simulink model "untitled1"  (R2022b)
settings: Solver=FixedStepDiscrete  StartTime=0.0  StopTime=1  FixedStep=1  RelTol=1e-3
settings Model: Creator=vanch  LastModifiedBy=vanch

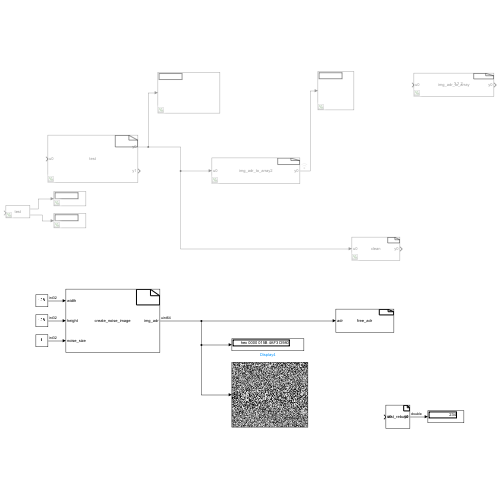
[thumbnail: Simulink's stored preview of the top-level diagram]
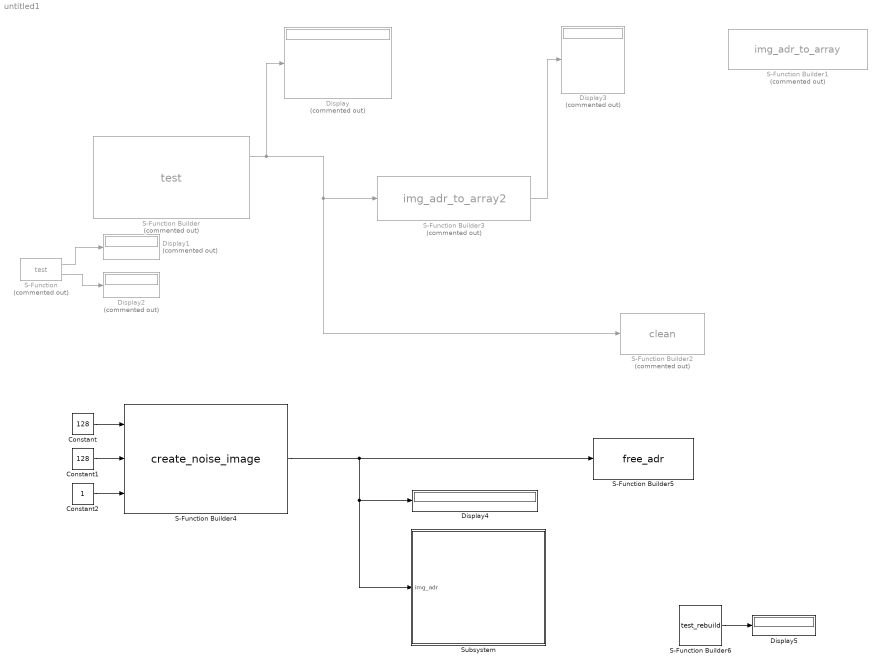
== system untitled1 ==
  Constant : Constant  Value=128  OutDataTypeStr=int32
  Constant1 : Constant  Value=128  OutDataTypeStr=int32
  Constant2 : Constant  OutDataTypeStr=int32
  Display{,1..3} (4 alike) : Display  Commented=on
      Display settings: Format=hex (Stored Integer)
  Display4 : Display
      settings: Format=hex (Stored Integer)
  Display5 : Display
  S-Function : S-Function  Commented=on  FunctionName=test  Parameters=3  SFunctionDeploymentMode=off  EnableBusSupport=off
  S-Function Builder : S-Function  Commented=on  FunctionName=test  Parameters=1  SFunctionModules=test_wrapper.cpp  SFunctionDeploymentMode=off  EnableBusSupport=off  mask(S-Function Builder){}
      mask help: Simulink:masks:SFunctionBuilder_MD
      mask init:
      | val = [[.9  0.75 0.75 1 1 .9 .9 1]',[1 1 0.75 0.75 .9 .9 1 .9]'];try , sys = get_param(gcb,'SfunBuilderFcnName');if isempty(sys), sys = get_param(gcb,'FunctionName'); end,catch, sys = get_param(gcb,'FunctionName'); end
      settings: CopyFcn=set_param(gcbh,'LinkStatus','none')  OpenFcn=sfunctionwizard(gcbh)
      mask Display:
      | plot(val(:,1),val(:,2))
      | disp(sys)
      | port_label('input',1,'u0')
      | port_label('output',1,'y0')
      | port_label('output',2,'y1')
  S-Function Builder1 : S-Function  Commented=on  FunctionName=img_adr_to_array  SFunctionModules=img_adr_to_array_wrapper.cpp  SFunctionDeploymentMode=off  EnableBusSupport=off  mask(S-Function Builder){}
      mask help: Simulink:masks:SFunctionBuilder_MD
      mask init: same as untitled1/S-Function Builder
      settings: CopyFcn=set_param(gcbh,'LinkStatus','none')  OpenFcn=sfunctionwizard(gcbh)
      mask Display: plot(val(:,1),val(:,2)),disp(sys),port_label('input',1,'u0'),port_label('output',1,'y0'),port_label('output',2,'y1')
  S-Function Builder2 : S-Function  Commented=on  FunctionName=clean  SFunctionModules=clean_wrapper.cpp  SFunctionDeploymentMode=off  EnableBusSupport=off  mask(S-Function Builder){}
      mask help: Simulink:masks:SFunctionBuilder_MD
      mask init: same as untitled1/S-Function Builder
      settings: CopyFcn=set_param(gcbh,'LinkStatus','none')  OpenFcn=sfunctionwizard(gcbh)
      mask Display:
      | plot(val(:,1),val(:,2))
      | disp(sys)
      | port_label('input',1,'u0')
      | port_label('output',1,'y0')
  S-Function Builder3 : S-Function  Commented=on  FunctionName=img_adr_to_array2  SFunctionModules=img_adr_to_array2_wrapper.cpp  SFunctionDeploymentMode=off  EnableBusSupport=off  mask(S-Function Builder){}
      mask help: Simulink:masks:SFunctionBuilder_MD
      mask init: same as untitled1/S-Function Builder
      settings: CopyFcn=set_param(gcbh,'LinkStatus','none')  OpenFcn=sfunctionwizard(gcbh)
      mask Display:
      | plot(val(:,1),val(:,2))
      | disp(sys)
      | port_label('input',1,'u0')
      | port_label('output',1,'y0')
  S-Function Builder4 : S-Function  FunctionName=create_noise_image  SFunctionModules=create_noise_image_wrapper.c  SFunctionDeploymentMode=off  EnableBusSupport=off  mask(S-Function Builder){}
      mask help: Simulink:masks:SFunctionBuilder_MD
      mask init: same as untitled1/S-Function Builder
      settings: CopyFcn=set_param(gcbh,'LinkStatus','none')  OpenFcn=sfunctionwizard(gcbh)
      mask Display:
      | plot(val(:,1),val(:,2))
      | disp(sys)
      | port_label('input',1,'width')
      | port_label('input',2,'height')
      | port_label('input',3,'noise_size')
      | port_label('output',1,'img_adr')
  S-Function Builder5 : S-Function  Priority=2  FunctionName=free_adr  SFunctionModules=free_adr_wrapper.c  SFunctionDeploymentMode=off  EnableBusSupport=off  mask(S-Function Builder){}
      mask help: Simulink:masks:SFunctionBuilder_MD
      mask init: same as untitled1/S-Function Builder
      settings: CopyFcn=set_param(gcbh,'LinkStatus','none')  OpenFcn=sfunctionwizard(gcbh)
      mask Display:
      | plot(val(:,1),val(:,2))
      | disp(sys)
      | port_label('input',1,'adr')
  S-Function Builder6 : S-Function  FunctionName=test_rebuild  SFunctionModules=test_rebuild_wrapper.c  SFunctionDeploymentMode=off  EnableBusSupport=off  mask(S-Function Builder){}
      mask help: Simulink:masks:SFunctionBuilder_MD
      mask init: same as untitled1/S-Function Builder
      settings: CopyFcn=set_param(gcbh,'LinkStatus','none')  OpenFcn=sfunctionwizard(gcbh)
      mask Display:
      | plot(val(:,1),val(:,2))
      | disp(sys)
      | port_label('input',1,'u0')
      | port_label('output',1,'y0')
  Subsystem : Subsystem  Priority=1  StopFcn=disp('stop')
      settings: PauseFcn=|
      | disp('paused')
      | %image('output.png')
      | disp(gcb)
      | maskobj = get_param(gcb, 'MaskObject')
      | maskobj.Display = char(string('image(''output.png'');')+"a="+string(rand()))
      | 
      | %set_param(gcb, 'MaskObject', maskobj)
      mask Display: image('output.png');a=0.81428
  wires:
  S-Function/1 -> Display1/1
  S-Function/2 -> Display2/1
  S-Function Builder3/1 -> Display3/1
  S-Function Builder/1 -> S-Function Builder3/1, S-Function Builder2/1, Display/1
  Constant/1 -> S-Function Builder4/1
  Constant1/1 -> S-Function Builder4/2
  S-Function Builder4/1 -> S-Function Builder5/1, Subsystem/1(img_adr), Display4/1
  Constant2/1 -> S-Function Builder4/3
  S-Function Builder6/1 -> Display5/1

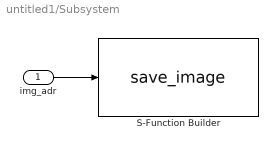
== system untitled1/Subsystem ==
  img_adr : Inport
  S-Function Builder : S-Function  FunctionName=save_image  SFunctionModules=save_image_wrapper.c  SFunctionDeploymentMode=off  EnableBusSupport=off  mask(S-Function Builder){}
      mask help: Simulink:masks:SFunctionBuilder_MD
      mask init: same as untitled1/S-Function Builder
      settings: CopyFcn=set_param(gcbh,'LinkStatus','none')  OpenFcn=sfunctionwizard(gcbh)
      mask Display:
      | plot(val(:,1),val(:,2))
      | disp(sys)
      | port_label('input',1,'img_adr')
  wires:
  img_adr/1 -> S-Function Builder/1
